simulink model "IK_Six_DOF_assembly2"  (R2022b)
settings: Solver=VariableStepAuto  StartTime=0.0  StopTime=500  RelTol=1e-3
model workspace: external: MATLAB File S:\project works\FYP\matlab\test2\6_DOF_assembly2\Assembly11_DataFile.m (data not in the file)
undefined symbols (not defined in the file or in its folder): sigbuilder_block, smiData, X, Y, Z
libraries: sm_lib x411, nesl_utility x45, slpidlib x14, robotcorelib x5, robotmaniplib x2
(part 2 of 9)

== system IK_Six_DOF_assembly2/Robot ==
  motion : Inport
  Calf Support Subsystem : Subsystem
  Initializer : Subsystem
  Subsystem : Subsystem
  Thigh/Slider Subsystem1 : Subsystem
  Thigh/Slider Subsystem2 : Subsystem
  qm : Outport
  wires:
  motion/1 -> Subsystem/1(motion)
  Subsystem/1(Position) -> qm/1  "qm"
  connections:
  Thigh/Slider Subsystem1/RConn1 -- Initializer/RConn1
  Calf Support Subsystem/LConn2 -- Thigh/Slider Subsystem2/LConn1
  Calf Support Subsystem/LConn1 -- Thigh/Slider Subsystem1/LConn1
  Subsystem/LConn1 -- Calf Support Subsystem/RConn1
  Subsystem/LConn2 -- Calf Support Subsystem/RConn2

== system IK_Six_DOF_assembly2/Robot1 ==
  torque : Inport
  Calf Support Subsystem : Subsystem
  Initializer : Subsystem
  Subsystem : Subsystem
  Thigh/Slider Subsystem1 : Subsystem
  Thigh/Slider Subsystem2 : Subsystem
  qm : Outport
  wires:
  Subsystem/1(Position) -> qm/1  "qm"
  torque/1 -> Subsystem/1(torque)
  connections:
  Subsystem/LConn2 -- Calf Support Subsystem/RConn2
  Subsystem/LConn1 -- Calf Support Subsystem/RConn1
  Calf Support Subsystem/LConn1 -- Thigh/Slider Subsystem1/LConn1
  Calf Support Subsystem/LConn2 -- Thigh/Slider Subsystem2/LConn1
  Thigh/Slider Subsystem1/RConn1 -- Initializer/RConn1

== system IK_Six_DOF_assembly2/Robot2 ==
  torque : Inport
  Calf Support Subsystem : Subsystem
  Initializer : Subsystem
  Subsystem : Subsystem
  Thigh/Slider Subsystem1 : Subsystem
  Thigh/Slider Subsystem2 : Subsystem
  qm : Outport
  wires:
  torque/1 -> Subsystem/1(torque)
  Subsystem/1(Position) -> qm/1  "qm"
  connections:
  Thigh/Slider Subsystem1/RConn1 -- Initializer/RConn1
  Calf Support Subsystem/LConn2 -- Thigh/Slider Subsystem2/LConn1
  Calf Support Subsystem/LConn1 -- Thigh/Slider Subsystem1/LConn1
  Subsystem/LConn1 -- Calf Support Subsystem/RConn1
  Subsystem/LConn2 -- Calf Support Subsystem/RConn2

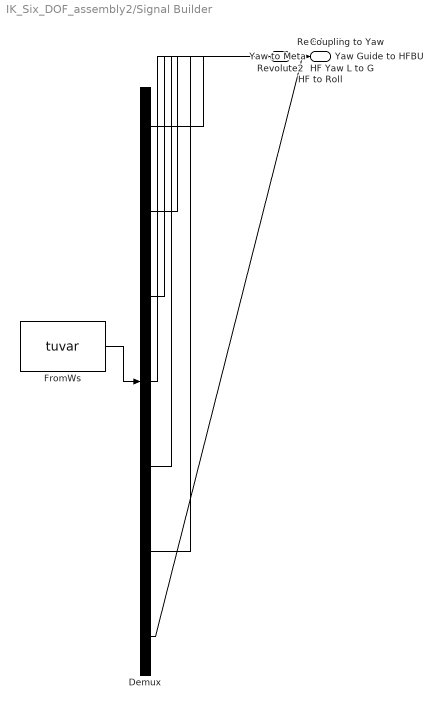
== system IK_Six_DOF_assembly2/Signal Builder ==
  Demux : Demux  Tag=STV Demux  Outputs=7
      settings: DisplayOption=none
  FromWs : FromWorkspace  Tag=STV FromWs  VariableName=tuvar
      SigBuilderData=|
      | common.afterFinalStr = 'Extrapolate'
      | common.sampleTime = 0
      | dataSet.timeRange = [0 10]
      | dataSet.name = 'Group 1'
      | sbobj.Groups.Name = 'Group 1'
      | sbobj.Groups.Signals(1).Name = 'Revolute2'
      | sbobj.Groups.Signals(1).XData = [0 3.5 3.5 6.52 6.52 10]
      | sbobj.Groups.Signals(1).YData = [0 0 0.4 0.4 0 0]
      | sbobj.Groups.Signals(2).Name = 'Revolute1'
      | sbobj.Groups.Signals(2).XData = [0 2.98 2.98 6.98 6.98 10]
      | sbobj.Groups.Signals(2).YData = [0 0 0.45 0.45 0 0]
      | sbobj.Groups.Signals(3).Name = 'HF Yaw L to G'
      | sbobj.Groups.Signals(3).XData = [0 2.5 2.5 7.62 7.62 10]
      | sbobj.Groups.Signals(3).YData = [0 0 0.3 0.3 0 0]
      | sbobj.Groups.Signals(4).Name = 'Yaw Guide to HFBU'
      | sbobj.Groups.Signals(4).XData = [0 2 2 8 8 10]
      | sbobj.Groups.Signals(4).YData = [0 0 0.4 0.4 0 0]
      | sbobj.Groups.Signals(5).Name = 'HF to Roll'
      | sbobj.Groups.Signals(5).XData = [0 1.46 1.46 8.6 8.6 10]
      | sbobj.Groups.Signals(5).YData = [0 0 0.35 0.35 0 0]
      | sbobj.Groups.Signals(6).Name = 'Yaw to Meta'
      | sbobj.Groups.Signals(6).XData = [0 1.02 1.02 9.04 9.04 10]
      | sbobj.Groups.Signals(6).YData = [0 0 0.2 0.2 0 0]
      | sbobj.Groups.Signals(7).Name = 'Coupling to Yaw'
      | sbobj.Groups.Signals(7).XData = [0 0.58 0.58 9.5 9.5 10]
      | sbobj.Groups.Signals(7).YData = [0 0 0.5 0.5 0 0]
  Revolute2 : Outport  Tag=STV Outport
  Revolute1 : Outport  Tag=STV Outport  Port=2
  HF Yaw L to G : Outport  Tag=STV Outport  Port=3
  Yaw Guide to HFBU : Outport  Tag=STV Outport  Port=4
  HF to Roll : Outport  Tag=STV Outport  Port=5
  Yaw to Meta : Outport  Tag=STV Outport  Port=6
  Coupling to Yaw : Outport  Tag=STV Outport  Port=7
  wires:
  FromWs/1 -> Demux/1
  Demux/1 -> Revolute2/1
  Demux/2 -> Revolute1/1
  Demux/3 -> HF Yaw L to G/1
  Demux/4 -> Yaw Guide to HFBU/1
  Demux/5 -> HF to Roll/1
  Demux/6 -> Yaw to Meta/1
  Demux/7 -> Coupling to Yaw/1

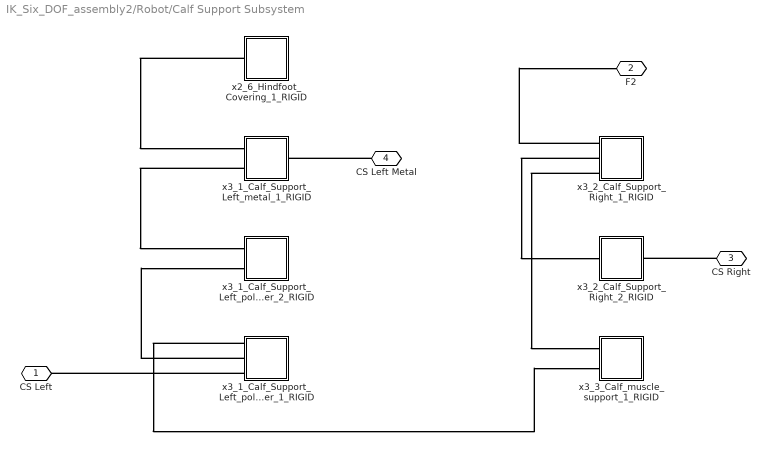
== system IK_Six_DOF_assembly2/Robot/Calf Support Subsystem ==
  x2_6_Hindfoot_Covering_1_RIGID : Subsystem
  x3_1_Calf_Support_Left_metal_1_RIGID : Subsystem
  x3_1_Calf_Support_Left_poly_upper_1_RIGID : Subsystem
  x3_1_Calf_Support_Left_poly_upper_2_RIGID : Subsystem
  x3_2_Calf_Support_Right_1_RIGID : Subsystem
  x3_2_Calf_Support_Right_2_RIGID : Subsystem
  x3_3_Calf_muscle_support_1_RIGID : Subsystem
  "CS Left " : PMIOPort  Side=Left
  F2 : PMIOPort  Port=2  Side=Left
  CS Right : PMIOPort  Port=3  Side=Right
  CS Left Metal : PMIOPort  Port=4  Side=Right
  connections:
  x2_6_Hindfoot_Covering_1_RIGID/LConn1 -- x3_1_Calf_Support_Left_metal_1_RIGID/LConn1
  x3_2_Calf_Support_Right_1_RIGID/LConn1 -- F2/RConn1
  x3_1_Calf_Support_Left_poly_upper_1_RIGID/LConn1 -- x3_3_Calf_muscle_support_1_RIGID/LConn2
  x3_2_Calf_Support_Right_1_RIGID/LConn2 -- x3_2_Calf_Support_Right_2_RIGID/LConn1
  CS Left Metal/RConn1 -- x3_1_Calf_Support_Left_metal_1_RIGID/RConn1
  x3_1_Calf_Support_Left_metal_1_RIGID/LConn2 -- x3_1_Calf_Support_Left_poly_upper_2_RIGID/LConn1
  x3_2_Calf_Support_Right_1_RIGID/LConn3 -- x3_3_Calf_muscle_support_1_RIGID/LConn1
  x3_1_Calf_Support_Left_poly_upper_1_RIGID/LConn2 -- x3_1_Calf_Support_Left_poly_upper_2_RIGID/LConn2
  CS Right/RConn1 -- x3_2_Calf_Support_Right_2_RIGID/RConn1
  x3_1_Calf_Support_Left_poly_upper_1_RIGID/LConn3 -- "CS Left "/RConn1

== system IK_Six_DOF_assembly2/Robot/Initializer ==
  MechanismConfiguration : sm_lib/Utilities/Mechanism Configuration  UniformGravity=Constant  GravityVector=[0 0 -9.80665]  GravityUnits=m/s^2  LinearizationDelta=0.001  JointModeTransitionNonlinearIterations=2
  Solver Configuration : nesl_utility/Solver Configuration  PhysicalDomain=network_engine_domain  SubClassName=solver  LeftPortType=input  RightPortType=generic  Tones=[]  Harmonics=[]  SimulateNoise=off  Profile=off  UseLocalSampling=off  EnableSwitchedLinearOptims=on  FrequencyDomain=off  UseCCode=off  RelTol=0.001  AbsTol=1e-06  MinStep=1e-09  ToWorkspace=off  RevertToSquareIcSolve=off  NumHomotopyIterations=100  PhasorMode=off  PhasorModeNumHarmonics=1  ConsistencySolver=NEWTON_FTOL  IndexReductionMethod=DerivativeReplacement  DoDC=off  ResidualTolerance=1e-09  ConsistencyTolSource=GLOBAL  ConsistencyAbsTol=0.001  ConsistencyRelTol=0.001  ConsistencyTolFactor=0.001  UseLocalSolver=off  LocalSolverChoice=NE_BACKWARD_EULER_ADVANCER  ResolveIndetEquations=on  FunctionEvalNumThread=1  LocalSolverSampleTime=0.001  DoFixedCost=off  MaxNonlinIter=3  MaxModeIter=2  ComputeImpulses=off  ImpulseIterations=2  LinearAlgebra=auto  LinearAlgebraNumThread=0  EquationFormulation=NE_TIME_EF  DelaysMemoryBudget=1024  AutomaticFiltering=on  FilteringTimeConstant=0.001  PartitionStorageMethod=AS_NEEDED  PartitionMemoryBudget=1024  PartitionMethod=ROBUST
  Transform : sm_lib/Frames and Transforms/Rigid Transform  TranslationMethod=Cartesian  TranslationStandardOffset=0  TranslationLengthUnit=in  TranslationStandardAxis=+Z  TranslationCartesianOffset=smiData.RigidTransform(63).translation  TranslationROffset=0  TranslationROffsetUnits=m  TranslationZOffset=0  TranslationZOffsetUnits=m  TranslationThetaOffset=0  TranslationThetaOffsetUnits=deg  RotationMethod=ArbitraryAxis  RotationAngleUnits=rad  RotationStandardAxis=+Z  RotationAngle=smiData.RigidTransform(63).angle  RotationArbitraryAxis=smiData.RigidTransform(63).axis  FollAlignAxisA=+X  BaseAlignAxisA=+Y  FollAlignAxisB=+Y  BaseAlignAxisB=+Z  RotationSequenceAxes=FollowerAxes  RotationSequence=XYX  RotationSequenceAngles=[0 0 0]  RotationSequenceAnglesUnits=deg  RotationMatrix=[1 0 0; 0 1 0; 0 0 1]  Quaternion=[1 0 0 0]
  World : sm_lib/Frames and Transforms/World Frame
  F2 : PMIOPort  Side=Right
  connections:
  Transform/LConn1 -- Solver Configuration/RConn1 -- MechanismConfiguration/RConn1 -- World/RConn1
  Transform/RConn1 -- F2/RConn1

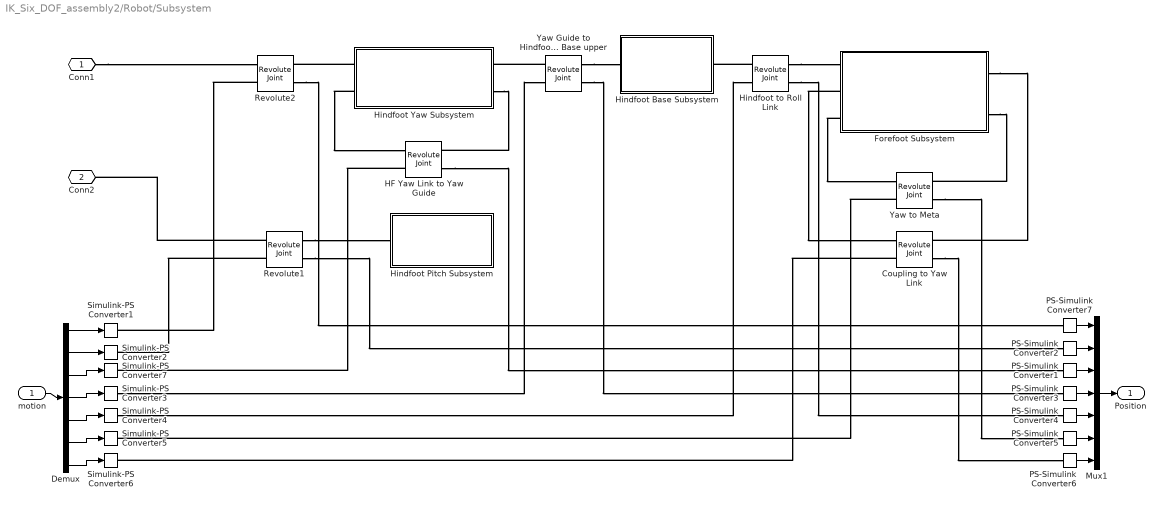
== system IK_Six_DOF_assembly2/Robot/Subsystem ==
  motion : Inport
  Coupling to Yaw Link : sm_lib/Joints/Revolute Joint  JointMode=Normal  SenseConstraintForce=off  SenseConstraintForceX=off  SenseConstraintForceY=off  SenseConstraintForceZ=off  SenseConstraintTorque=off  SenseConstraintTorqueX=off  SenseConstraintTorqueY=off  SenseConstraintTorqueZ=off  SenseTotalForce=off  SenseTotalForceX=off  SenseTotalForceY=off  SenseTotalForceZ=off  SenseTotalTorque=off  SenseTotalTorqueX=off  SenseTotalTorqueY=off  SenseTotalTorqueZ=off  CompositeWrenchDir=FollowerOnBase  CompositeWrenchFrame=BaseFrame  EquilibriumPosition=0  EquilibriumPositionUnits=deg  SpringStiffness=0  SpringStiffnessUnits=N*m/deg  DampingCoefficient=0  DampingCoefficientUnits=N*m/(deg/s)  TorqueActuationMode=ComputedTorque  MotionActuationMode=InputMotion  SensePosition=on  SenseVelocity=off  SenseAcceleration=off  SenseTorqueForce=off  SenseLowerLimitTorqueForce=off  SenseUpperLimitTorqueForce=off  LowerLimitSpecify=off  LowerLimitBound=-90  LowerLimitBoundUnits=deg  LowerLimitStiffness=1e4  LowerLimitStiffnessUnits=N*m/deg  LowerLimitDamping=10  LowerLimitDampingUnits=N*m/(deg/s)  LowerLimitTransitionRegionWidth=0.1  LowerLimitTransitionRegionWidthUnits=deg  UpperLimitSpecify=off  UpperLimitBound=90  UpperLimitBoundUnits=deg  UpperLimitStiffness=1e4  UpperLimitStiffnessUnits=N*m/deg  UpperLimitDamping=10  UpperLimitDampingUnits=N*m/(deg/s)  UpperLimitTransitionRegionWidth=0.1  UpperLimitTransitionRegionWidthUnits=deg  PositionTargetSpecify=on  PositionTargetPriority=Low  PositionTargetValue=smiData.RevoluteJoint(7).Rz.Pos  PositionTargetValueUnits=deg  VelocityTargetSpecify=off  VelocityTargetPriority=High  VelocityTargetValue=0  VelocityTargetValueUnits=deg/s
  Demux : Demux  Outputs=7
  Forefoot Subsystem : Subsystem
  HF Yaw Link to Yaw Guide : sm_lib/Joints/Revolute Joint  JointMode=Normal  SenseConstraintForce=off  SenseConstraintForceX=off  SenseConstraintForceY=off  SenseConstraintForceZ=off  SenseConstraintTorque=off  SenseConstraintTorqueX=off  SenseConstraintTorqueY=off  SenseConstraintTorqueZ=off  SenseTotalForce=off  SenseTotalForceX=off  SenseTotalForceY=off  SenseTotalForceZ=off  SenseTotalTorque=off  SenseTotalTorqueX=off  SenseTotalTorqueY=off  SenseTotalTorqueZ=off  CompositeWrenchDir=FollowerOnBase  CompositeWrenchFrame=BaseFrame  EquilibriumPosition=0  EquilibriumPositionUnits=deg  SpringStiffness=0  SpringStiffnessUnits=N*m/deg  DampingCoefficient=0  DampingCoefficientUnits=N*m/(deg/s)  TorqueActuationMode=ComputedTorque  MotionActuationMode=InputMotion  SensePosition=on  SenseVelocity=off  SenseAcceleration=off  SenseTorqueForce=off  SenseLowerLimitTorqueForce=off  SenseUpperLimitTorqueForce=off  LowerLimitSpecify=off  LowerLimitBound=-30  LowerLimitBoundUnits=deg  LowerLimitStiffness=1e4  LowerLimitStiffnessUnits=N*m/deg  LowerLimitDamping=10  LowerLimitDampingUnits=N*m/(deg/s)  LowerLimitTransitionRegionWidth=0.1  LowerLimitTransitionRegionWidthUnits=deg  UpperLimitSpecify=off  UpperLimitBound=30  UpperLimitBoundUnits=deg  UpperLimitStiffness=1e4  UpperLimitStiffnessUnits=N*m/deg  UpperLimitDamping=10  UpperLimitDampingUnits=N*m/(deg/s)  UpperLimitTransitionRegionWidth=0.1  UpperLimitTransitionRegionWidthUnits=deg  PositionTargetSpecify=on  PositionTargetPriority=Low  PositionTargetValue=smiData.RevoluteJoint(2).Rz.Pos  PositionTargetValueUnits=deg  VelocityTargetSpecify=off  VelocityTargetPriority=High  VelocityTargetValue=0  VelocityTargetValueUnits=deg/s
  Hindfoot Base Subsystem : Subsystem
  Hindfoot Pitch Subsystem : Subsystem
  Hindfoot Yaw Subsystem : Subsystem
  Hindfoot to Roll Link : sm_lib/Joints/Revolute Joint  JointMode=Normal  SenseConstraintForce=off  SenseConstraintForceX=off  SenseConstraintForceY=off  SenseConstraintForceZ=off  SenseConstraintTorque=off  SenseConstraintTorqueX=off  SenseConstraintTorqueY=off  SenseConstraintTorqueZ=off  SenseTotalForce=off  SenseTotalForceX=off  SenseTotalForceY=off  SenseTotalForceZ=off  SenseTotalTorque=off  SenseTotalTorqueX=off  SenseTotalTorqueY=off  SenseTotalTorqueZ=off  CompositeWrenchDir=FollowerOnBase  CompositeWrenchFrame=BaseFrame  EquilibriumPosition=0  EquilibriumPositionUnits=deg  SpringStiffness=0  SpringStiffnessUnits=N*m/deg  DampingCoefficient=0  DampingCoefficientUnits=N*m/(deg/s)  TorqueActuationMode=ComputedTorque  MotionActuationMode=InputMotion  SensePosition=on  SenseVelocity=off  SenseAcceleration=off  SenseTorqueForce=off  SenseLowerLimitTorqueForce=off  SenseUpperLimitTorqueForce=off  LowerLimitSpecify=off  LowerLimitBound=-90  LowerLimitBoundUnits=deg  LowerLimitStiffness=1e4  LowerLimitStiffnessUnits=N*m/deg  LowerLimitDamping=10  LowerLimitDampingUnits=N*m/(deg/s)  LowerLimitTransitionRegionWidth=0.1  LowerLimitTransitionRegionWidthUnits=deg  UpperLimitSpecify=off  UpperLimitBound=90  UpperLimitBoundUnits=deg  UpperLimitStiffness=1e4  UpperLimitStiffnessUnits=N*m/deg  UpperLimitDamping=10  UpperLimitDampingUnits=N*m/(deg/s)  UpperLimitTransitionRegionWidth=0.1  UpperLimitTransitionRegionWidthUnits=deg  PositionTargetSpecify=on  PositionTargetPriority=Low  PositionTargetValue=smiData.RevoluteJoint(6).Rz.Pos  PositionTargetValueUnits=deg  VelocityTargetSpecify=off  VelocityTargetPriority=High  VelocityTargetValue=0  VelocityTargetValueUnits=deg/s
  Mux1 : Mux  Inputs=7
  PS-Simulink Converter{1..7} (7 alike) : nesl_utility/PS-Simulink Converter  PhysicalDomain=network_engine_domain  SubClassName=ps_output  LeftPortType=input  RightPortType=output  PseudoPeriodic=off  Frequencies=[]  VectorFormat=1-D array  Unit=inherit  AffineConversion=off
  Revolute1 : sm_lib/Joints/Revolute Joint  JointMode=Normal  SenseConstraintForce=off  SenseConstraintForceX=off  SenseConstraintForceY=off  SenseConstraintForceZ=off  SenseConstraintTorque=off  SenseConstraintTorqueX=off  SenseConstraintTorqueY=off  SenseConstraintTorqueZ=off  SenseTotalForce=off  SenseTotalForceX=off  SenseTotalForceY=off  SenseTotalForceZ=off  SenseTotalTorque=off  SenseTotalTorqueX=off  SenseTotalTorqueY=off  SenseTotalTorqueZ=off  CompositeWrenchDir=FollowerOnBase  CompositeWrenchFrame=BaseFrame  EquilibriumPosition=0  EquilibriumPositionUnits=deg  SpringStiffness=0  SpringStiffnessUnits=N*m/deg  DampingCoefficient=0  DampingCoefficientUnits=N*m/(deg/s)  TorqueActuationMode=ComputedTorque  MotionActuationMode=InputMotion  SensePosition=on  SenseVelocity=off  SenseAcceleration=off  SenseTorqueForce=off  SenseLowerLimitTorqueForce=off  SenseUpperLimitTorqueForce=off  LowerLimitSpecify=off  LowerLimitBound=-25  LowerLimitBoundUnits=deg  LowerLimitStiffness=1e4  LowerLimitStiffnessUnits=N*m/deg  LowerLimitDamping=10  LowerLimitDampingUnits=N*m/(deg/s)  LowerLimitTransitionRegionWidth=0.1  LowerLimitTransitionRegionWidthUnits=deg  UpperLimitSpecify=off  UpperLimitBound=25  UpperLimitBoundUnits=deg  UpperLimitStiffness=1e4  UpperLimitStiffnessUnits=N*m/deg  UpperLimitDamping=10  UpperLimitDampingUnits=N*m/(deg/s)  UpperLimitTransitionRegionWidth=0.1  UpperLimitTransitionRegionWidthUnits=deg  PositionTargetSpecify=on  PositionTargetPriority=Low  PositionTargetValue=smiData.RevoluteJoint(4).Rz.Pos  PositionTargetValueUnits=deg  VelocityTargetSpecify=off  VelocityTargetPriority=High  VelocityTargetValue=0  VelocityTargetValueUnits=deg/s
  Revolute2 : sm_lib/Joints/Revolute Joint  JointMode=Normal  SenseConstraintForce=off  SenseConstraintForceX=off  SenseConstraintForceY=off  SenseConstraintForceZ=off  SenseConstraintTorque=off  SenseConstraintTorqueX=off  SenseConstraintTorqueY=off  SenseConstraintTorqueZ=off  SenseTotalForce=off  SenseTotalForceX=off  SenseTotalForceY=off  SenseTotalForceZ=off  SenseTotalTorque=off  SenseTotalTorqueX=off  SenseTotalTorqueY=off  SenseTotalTorqueZ=off  CompositeWrenchDir=FollowerOnBase  CompositeWrenchFrame=BaseFrame  EquilibriumPosition=0  EquilibriumPositionUnits=deg  SpringStiffness=0  SpringStiffnessUnits=N*m/deg  DampingCoefficient=0  DampingCoefficientUnits=N*m/(deg/s)  TorqueActuationMode=ComputedTorque  MotionActuationMode=InputMotion  SensePosition=on  SenseVelocity=off  SenseAcceleration=off  SenseTorqueForce=off  SenseLowerLimitTorqueForce=off  SenseUpperLimitTorqueForce=off  LowerLimitSpecify=off  LowerLimitBound=-25  LowerLimitBoundUnits=deg  LowerLimitStiffness=1e4  LowerLimitStiffnessUnits=N*m/deg  LowerLimitDamping=10  LowerLimitDampingUnits=N*m/(deg/s)  LowerLimitTransitionRegionWidth=0.1  LowerLimitTransitionRegionWidthUnits=deg  UpperLimitSpecify=off  UpperLimitBound=25  UpperLimitBoundUnits=deg  UpperLimitStiffness=1e4  UpperLimitStiffnessUnits=N*m/deg  UpperLimitDamping=10  UpperLimitDampingUnits=N*m/(deg/s)  UpperLimitTransitionRegionWidth=0.1  UpperLimitTransitionRegionWidthUnits=deg  PositionTargetSpecify=on  PositionTargetPriority=Low  PositionTargetValue=smiData.RevoluteJoint(4).Rz.Pos  PositionTargetValueUnits=deg  VelocityTargetSpecify=off  VelocityTargetPriority=High  VelocityTargetValue=0  VelocityTargetValueUnits=deg/s
  Simulink-PS Converter{1..7} (7 alike) : nesl_utility/Simulink-PS Converter  PhysicalDomain=network_engine_domain  SubClassName=ps_input  LeftPortType=input  RightPortType=output  PseudoPeriodic=off  Frequencies=[]  NoiseDistribution=none  NoiseParameters=[]  Unit=rad  AffineConversion=off  FilteringAndDerivatives=filter  SimscapeFilterOrder=2  InputFilterTimeConstant=0.001  UdotUserProvided=0
  Yaw Guide to Hindfoot Base upper : sm_lib/Joints/Revolute Joint  JointMode=Normal  SenseConstraintForce=off  SenseConstraintForceX=off  SenseConstraintForceY=off  SenseConstraintForceZ=off  SenseConstraintTorque=off  SenseConstraintTorqueX=off  SenseConstraintTorqueY=off  SenseConstraintTorqueZ=off  SenseTotalForce=off  SenseTotalForceX=off  SenseTotalForceY=off  SenseTotalForceZ=off  SenseTotalTorque=off  SenseTotalTorqueX=off  SenseTotalTorqueY=off  SenseTotalTorqueZ=off  CompositeWrenchDir=FollowerOnBase  CompositeWrenchFrame=BaseFrame  EquilibriumPosition=0  EquilibriumPositionUnits=deg  SpringStiffness=0  SpringStiffnessUnits=N*m/deg  DampingCoefficient=0  DampingCoefficientUnits=N*m/(deg/s)  TorqueActuationMode=ComputedTorque  MotionActuationMode=InputMotion  SensePosition=on  SenseVelocity=off  SenseAcceleration=off  SenseTorqueForce=off  SenseLowerLimitTorqueForce=off  SenseUpperLimitTorqueForce=off  LowerLimitSpecify=off  LowerLimitBound=-90  LowerLimitBoundUnits=deg  LowerLimitStiffness=1e4  LowerLimitStiffnessUnits=N*m/deg  LowerLimitDamping=10  LowerLimitDampingUnits=N*m/(deg/s)  LowerLimitTransitionRegionWidth=0.1  LowerLimitTransitionRegionWidthUnits=deg  UpperLimitSpecify=off  UpperLimitBound=90  UpperLimitBoundUnits=deg  UpperLimitStiffness=1e4  UpperLimitStiffnessUnits=N*m/deg  UpperLimitDamping=10  UpperLimitDampingUnits=N*m/(deg/s)  UpperLimitTransitionRegionWidth=0.1  UpperLimitTransitionRegionWidthUnits=deg  PositionTargetSpecify=on  PositionTargetPriority=Low  PositionTargetValue=smiData.RevoluteJoint(3).Rz.Pos  PositionTargetValueUnits=deg  VelocityTargetSpecify=off  VelocityTargetPriority=High  VelocityTargetValue=0  VelocityTargetValueUnits=deg/s
  Yaw to Meta : sm_lib/Joints/Revolute Joint  JointMode=Normal  SenseConstraintForce=off  SenseConstraintForceX=off  SenseConstraintForceY=off  SenseConstraintForceZ=off  SenseConstraintTorque=off  SenseConstraintTorqueX=off  SenseConstraintTorqueY=off  SenseConstraintTorqueZ=off  SenseTotalForce=off  SenseTotalForceX=off  SenseTotalForceY=off  SenseTotalForceZ=off  SenseTotalTorque=off  SenseTotalTorqueX=off  SenseTotalTorqueY=off  SenseTotalTorqueZ=off  CompositeWrenchDir=FollowerOnBase  CompositeWrenchFrame=BaseFrame  EquilibriumPosition=0  EquilibriumPositionUnits=deg  SpringStiffness=0  SpringStiffnessUnits=N*m/deg  DampingCoefficient=0  DampingCoefficientUnits=N*m/(deg/s)  TorqueActuationMode=ComputedTorque  MotionActuationMode=InputMotion  SensePosition=on  SenseVelocity=off  SenseAcceleration=off  SenseTorqueForce=off  SenseLowerLimitTorqueForce=off  SenseUpperLimitTorqueForce=off  LowerLimitSpecify=off  LowerLimitBound=-90  LowerLimitBoundUnits=deg  LowerLimitStiffness=1e4  LowerLimitStiffnessUnits=N*m/deg  LowerLimitDamping=10  LowerLimitDampingUnits=N*m/(deg/s)  LowerLimitTransitionRegionWidth=0.1  LowerLimitTransitionRegionWidthUnits=deg  UpperLimitSpecify=off  UpperLimitBound=90  UpperLimitBoundUnits=deg  UpperLimitStiffness=1e4  UpperLimitStiffnessUnits=N*m/deg  UpperLimitDamping=10  UpperLimitDampingUnits=N*m/(deg/s)  UpperLimitTransitionRegionWidth=0.1  UpperLimitTransitionRegionWidthUnits=deg  PositionTargetSpecify=on  PositionTargetPriority=Low  PositionTargetValue=smiData.RevoluteJoint(5).Rz.Pos  PositionTargetValueUnits=deg  VelocityTargetSpecify=off  VelocityTargetPriority=High  VelocityTargetValue=0  VelocityTargetValueUnits=deg/s
  Conn1 : PMIOPort  Side=Left
  Conn2 : PMIOPort  Port=2  Side=Left
  Position : Outport
  wires:
  motion/1 -> Demux/1
  Demux/6 -> Simulink-PS Converter5/1
  Mux1/1 -> Position/1
  Demux/5 -> Simulink-PS Converter4/1
  Demux/7 -> Simulink-PS Converter6/1
  Demux/4 -> Simulink-PS Converter3/1
  PS-Simulink Converter3/1 -> Mux1/4
  PS-Simulink Converter4/1 -> Mux1/5
  PS-Simulink Converter5/1 -> Mux1/6
  PS-Simulink Converter6/1 -> Mux1/7
  Demux/1 -> Simulink-PS Converter1/1
  Demux/2 -> Simulink-PS Converter2/1
  Demux/3 -> Simulink-PS Converter7/1
  PS-Simulink Converter7/1 -> Mux1/1
  PS-Simulink Converter2/1 -> Mux1/2
  PS-Simulink Converter1/1 -> Mux1/3
  connections:
  Yaw Guide to Hindfoot Base upper/LConn1 -- Hindfoot Yaw Subsystem/RConn1
  Yaw Guide to Hindfoot Base upper/RConn1 -- Hindfoot Base Subsystem/LConn1
  Hindfoot to Roll Link/RConn2 -- PS-Simulink Converter4/LConn1
  Hindfoot to Roll Link/LConn1 -- Hindfoot Base Subsystem/RConn1
  Hindfoot to Roll Link/RConn1 -- Forefoot Subsystem/LConn1
  Revolute1/RConn1 -- Hindfoot Pitch Subsystem/LConn1
  Conn1/RConn1 -- Revolute2/LConn1
  Hindfoot Yaw Subsystem/RConn2 -- HF Yaw Link to Yaw Guide/RConn1
  Hindfoot Yaw Subsystem/LConn2 -- HF Yaw Link to Yaw Guide/LConn1
  Forefoot Subsystem/RConn2 -- Yaw to Meta/RConn1
  Yaw to Meta/LConn2 -- Simulink-PS Converter5/RConn1
  Forefoot Subsystem/LConn2 -- Coupling to Yaw Link/LConn1
  Revolute1/LConn1 -- Conn2/RConn1
  Coupling to Yaw Link/LConn2 -- Simulink-PS Converter6/RConn1
  Coupling to Yaw Link/RConn2 -- PS-Simulink Converter6/LConn1
  Yaw to Meta/RConn2 -- PS-Simulink Converter5/LConn1
  Simulink-PS Converter4/RConn1 -- Hindfoot to Roll Link/LConn2
  Forefoot Subsystem/RConn1 -- Coupling to Yaw Link/RConn1
  Forefoot Subsystem/LConn3 -- Yaw to Meta/LConn1
  Yaw Guide to Hindfoot Base upper/RConn2 -- PS-Simulink Converter3/LConn1
  Simulink-PS Converter3/RConn1 -- Yaw Guide to Hindfoot Base upper/LConn2
  Hindfoot Yaw Subsystem/LConn1 -- Revolute2/RConn1
  Revolute2/LConn2 -- Simulink-PS Converter1/RConn1
  Revolute1/LConn2 -- Simulink-PS Converter2/RConn1
  HF Yaw Link to Yaw Guide/LConn2 -- Simulink-PS Converter7/RConn1
  Revolute2/RConn2 -- PS-Simulink Converter7/LConn1
  Revolute1/RConn2 -- PS-Simulink Converter2/LConn1
  HF Yaw Link to Yaw Guide/RConn2 -- PS-Simulink Converter1/LConn1

== system IK_Six_DOF_assembly2/Robot/Thigh//Slider Subsystem1 ==
  x4_1_Slider_Link_1_RIGID : Subsystem
  x4_3_Thigh_Link_1_RIGID : Subsystem
  F1 : PMIOPort  Side=Left
  F2 : PMIOPort  Port=2  Side=Right
  connections:
  x4_1_Slider_Link_1_RIGID/LConn3 -- x4_3_Thigh_Link_1_RIGID/LConn1
  F1/RConn1 -- x4_1_Slider_Link_1_RIGID/LConn1
  F2/RConn1 -- x4_1_Slider_Link_1_RIGID/LConn2

== system IK_Six_DOF_assembly2/Robot/Thigh//Slider Subsystem2 ==
  x4_1_Slider_Link_2_RIGID : Subsystem
  x4_3_Thigh_Link_2_RIGID : Subsystem
  F : PMIOPort  Side=Left
  connections:
  x4_1_Slider_Link_2_RIGID/LConn1 -- x4_3_Thigh_Link_2_RIGID/LConn1
  F/RConn1 -- x4_1_Slider_Link_2_RIGID/LConn2

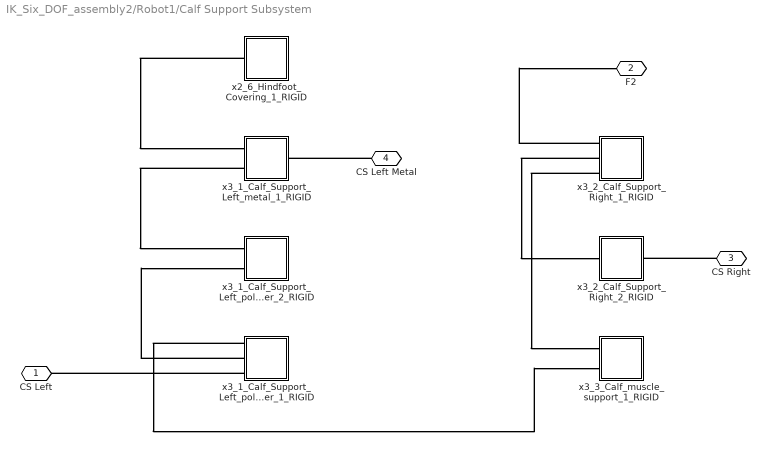
== system IK_Six_DOF_assembly2/Robot1/Calf Support Subsystem ==
  x2_6_Hindfoot_Covering_1_RIGID : Subsystem
  x3_1_Calf_Support_Left_metal_1_RIGID : Subsystem
  x3_1_Calf_Support_Left_poly_upper_1_RIGID : Subsystem
  x3_1_Calf_Support_Left_poly_upper_2_RIGID : Subsystem
  x3_2_Calf_Support_Right_1_RIGID : Subsystem
  x3_2_Calf_Support_Right_2_RIGID : Subsystem
  x3_3_Calf_muscle_support_1_RIGID : Subsystem
  "CS Left " : PMIOPort  Side=Left
  F2 : PMIOPort  Port=2  Side=Left
  CS Right : PMIOPort  Port=3  Side=Right
  CS Left Metal : PMIOPort  Port=4  Side=Right
  connections:
  x3_1_Calf_Support_Left_poly_upper_1_RIGID/LConn3 -- "CS Left "/RConn1
  CS Right/RConn1 -- x3_2_Calf_Support_Right_2_RIGID/RConn1
  x3_1_Calf_Support_Left_poly_upper_1_RIGID/LConn2 -- x3_1_Calf_Support_Left_poly_upper_2_RIGID/LConn2
  x3_2_Calf_Support_Right_1_RIGID/LConn3 -- x3_3_Calf_muscle_support_1_RIGID/LConn1
  x3_1_Calf_Support_Left_metal_1_RIGID/LConn2 -- x3_1_Calf_Support_Left_poly_upper_2_RIGID/LConn1
  CS Left Metal/RConn1 -- x3_1_Calf_Support_Left_metal_1_RIGID/RConn1
  x3_2_Calf_Support_Right_1_RIGID/LConn2 -- x3_2_Calf_Support_Right_2_RIGID/LConn1
  x3_1_Calf_Support_Left_poly_upper_1_RIGID/LConn1 -- x3_3_Calf_muscle_support_1_RIGID/LConn2
  x3_2_Calf_Support_Right_1_RIGID/LConn1 -- F2/RConn1
  x2_6_Hindfoot_Covering_1_RIGID/LConn1 -- x3_1_Calf_Support_Left_metal_1_RIGID/LConn1

== system IK_Six_DOF_assembly2/Robot1/Initializer ==
  MechanismConfiguration : sm_lib/Utilities/Mechanism Configuration  UniformGravity=Constant  GravityVector=[0 0 -9.80665]  GravityUnits=m/s^2  LinearizationDelta=0.001  JointModeTransitionNonlinearIterations=2
  Solver Configuration : nesl_utility/Solver Configuration  PhysicalDomain=network_engine_domain  SubClassName=solver  LeftPortType=input  RightPortType=generic  Tones=[]  Harmonics=[]  SimulateNoise=off  Profile=off  UseLocalSampling=off  EnableSwitchedLinearOptims=on  FrequencyDomain=off  UseCCode=off  RelTol=0.001  AbsTol=1e-06  MinStep=1e-09  ToWorkspace=off  RevertToSquareIcSolve=off  NumHomotopyIterations=100  PhasorMode=off  PhasorModeNumHarmonics=1  ConsistencySolver=NEWTON_FTOL  IndexReductionMethod=DerivativeReplacement  DoDC=off  ResidualTolerance=1e-09  ConsistencyTolSource=GLOBAL  ConsistencyAbsTol=0.001  ConsistencyRelTol=0.001  ConsistencyTolFactor=0.001  UseLocalSolver=off  LocalSolverChoice=NE_BACKWARD_EULER_ADVANCER  ResolveIndetEquations=on  FunctionEvalNumThread=1  LocalSolverSampleTime=0.001  DoFixedCost=off  MaxNonlinIter=3  MaxModeIter=2  ComputeImpulses=off  ImpulseIterations=2  LinearAlgebra=auto  LinearAlgebraNumThread=0  EquationFormulation=NE_TIME_EF  DelaysMemoryBudget=1024  AutomaticFiltering=on  FilteringTimeConstant=0.001  PartitionStorageMethod=AS_NEEDED  PartitionMemoryBudget=1024  PartitionMethod=ROBUST
  Transform : sm_lib/Frames and Transforms/Rigid Transform  TranslationMethod=Cartesian  TranslationStandardOffset=0  TranslationLengthUnit=in  TranslationStandardAxis=+Z  TranslationCartesianOffset=smiData.RigidTransform(63).translation  TranslationROffset=0  TranslationROffsetUnits=m  TranslationZOffset=0  TranslationZOffsetUnits=m  TranslationThetaOffset=0  TranslationThetaOffsetUnits=deg  RotationMethod=ArbitraryAxis  RotationAngleUnits=rad  RotationStandardAxis=+Z  RotationAngle=smiData.RigidTransform(63).angle  RotationArbitraryAxis=smiData.RigidTransform(63).axis  FollAlignAxisA=+X  BaseAlignAxisA=+Y  FollAlignAxisB=+Y  BaseAlignAxisB=+Z  RotationSequenceAxes=FollowerAxes  RotationSequence=XYX  RotationSequenceAngles=[0 0 0]  RotationSequenceAnglesUnits=deg  RotationMatrix=[1 0 0; 0 1 0; 0 0 1]  Quaternion=[1 0 0 0]
  World : sm_lib/Frames and Transforms/World Frame
  F2 : PMIOPort  Side=Right
  connections:
  Transform/RConn1 -- F2/RConn1
  World/RConn1 -- MechanismConfiguration/RConn1 -- Solver Configuration/RConn1 -- Transform/LConn1

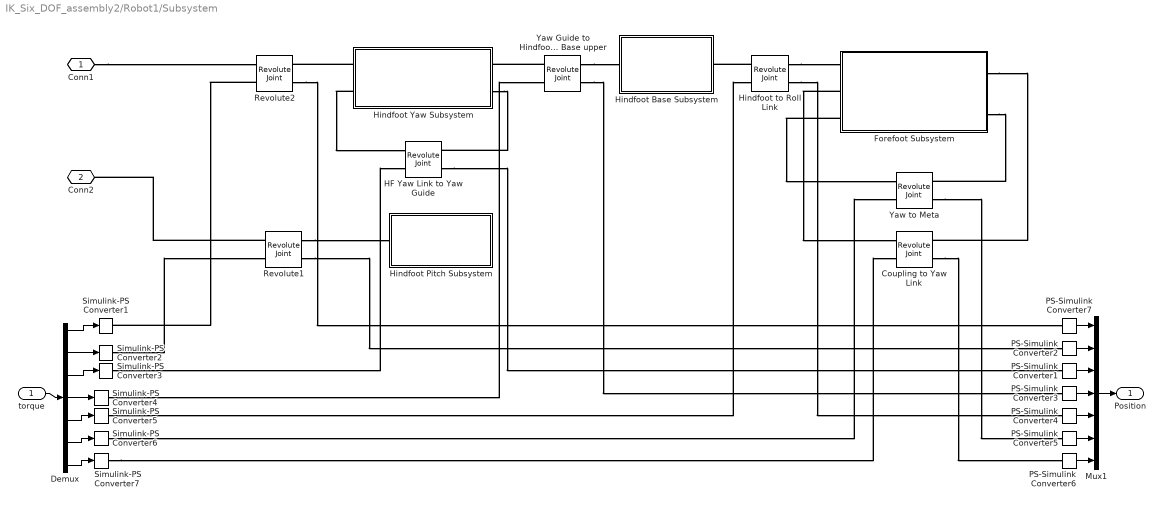
== system IK_Six_DOF_assembly2/Robot1/Subsystem ==
  torque : Inport
  Coupling to Yaw Link : sm_lib/Joints/Revolute Joint  JointMode=Normal  SenseConstraintForce=off  SenseConstraintForceX=off  SenseConstraintForceY=off  SenseConstraintForceZ=off  SenseConstraintTorque=off  SenseConstraintTorqueX=off  SenseConstraintTorqueY=off  SenseConstraintTorqueZ=off  SenseTotalForce=off  SenseTotalForceX=off  SenseTotalForceY=off  SenseTotalForceZ=off  SenseTotalTorque=off  SenseTotalTorqueX=off  SenseTotalTorqueY=off  SenseTotalTorqueZ=off  CompositeWrenchDir=FollowerOnBase  CompositeWrenchFrame=BaseFrame  EquilibriumPosition=0  EquilibriumPositionUnits=deg  SpringStiffness=0  SpringStiffnessUnits=N*m/deg  DampingCoefficient=0  DampingCoefficientUnits=N*m/(deg/s)  TorqueActuationMode=InputTorque  MotionActuationMode=ComputedMotion  SensePosition=on  SenseVelocity=off  SenseAcceleration=off  SenseTorqueForce=off  SenseLowerLimitTorqueForce=off  SenseUpperLimitTorqueForce=off  LowerLimitSpecify=on  LowerLimitBound=-25  LowerLimitBoundUnits=deg  LowerLimitStiffness=1e4  LowerLimitStiffnessUnits=N*m/deg  LowerLimitDamping=10  LowerLimitDampingUnits=N*m/(deg/s)  LowerLimitTransitionRegionWidth=0.1  LowerLimitTransitionRegionWidthUnits=deg  UpperLimitSpecify=on  UpperLimitBound=25  UpperLimitBoundUnits=deg  UpperLimitStiffness=1e4  UpperLimitStiffnessUnits=N*m/deg  UpperLimitDamping=10  UpperLimitDampingUnits=N*m/(deg/s)  UpperLimitTransitionRegionWidth=0.1  UpperLimitTransitionRegionWidthUnits=deg  PositionTargetSpecify=on  PositionTargetPriority=Low  PositionTargetValue=smiData.RevoluteJoint(7).Rz.Pos  PositionTargetValueUnits=deg  VelocityTargetSpecify=off  VelocityTargetPriority=High  VelocityTargetValue=0  VelocityTargetValueUnits=deg/s
  Demux : Demux  Outputs=7
  Forefoot Subsystem : Subsystem
  HF Yaw Link to Yaw Guide : sm_lib/Joints/Revolute Joint  JointMode=Normal  SenseConstraintForce=off  SenseConstraintForceX=off  SenseConstraintForceY=off  SenseConstraintForceZ=off  SenseConstraintTorque=off  SenseConstraintTorqueX=off  SenseConstraintTorqueY=off  SenseConstraintTorqueZ=off  SenseTotalForce=off  SenseTotalForceX=off  SenseTotalForceY=off  SenseTotalForceZ=off  SenseTotalTorque=off  SenseTotalTorqueX=off  SenseTotalTorqueY=off  SenseTotalTorqueZ=off  CompositeWrenchDir=FollowerOnBase  CompositeWrenchFrame=BaseFrame  EquilibriumPosition=0  EquilibriumPositionUnits=deg  SpringStiffness=0  SpringStiffnessUnits=N*m/deg  DampingCoefficient=0  DampingCoefficientUnits=N*m/(deg/s)  TorqueActuationMode=InputTorque  MotionActuationMode=ComputedMotion  SensePosition=on  SenseVelocity=off  SenseAcceleration=off  SenseTorqueForce=off  SenseLowerLimitTorqueForce=off  SenseUpperLimitTorqueForce=off  LowerLimitSpecify=on  LowerLimitBound=-30  LowerLimitBoundUnits=deg  LowerLimitStiffness=1e4  LowerLimitStiffnessUnits=N*m/deg  LowerLimitDamping=10  LowerLimitDampingUnits=N*m/(deg/s)  LowerLimitTransitionRegionWidth=0.1  LowerLimitTransitionRegionWidthUnits=deg  UpperLimitSpecify=on  UpperLimitBound=30  UpperLimitBoundUnits=deg  UpperLimitStiffness=1e4  UpperLimitStiffnessUnits=N*m/deg  UpperLimitDamping=10  UpperLimitDampingUnits=N*m/(deg/s)  UpperLimitTransitionRegionWidth=0.1  UpperLimitTransitionRegionWidthUnits=deg  PositionTargetSpecify=on  PositionTargetPriority=Low  PositionTargetValue=smiData.RevoluteJoint(2).Rz.Pos  PositionTargetValueUnits=deg  VelocityTargetSpecify=off  VelocityTargetPriority=High  VelocityTargetValue=0  VelocityTargetValueUnits=deg/s
  Hindfoot Base Subsystem : Subsystem
  Hindfoot Pitch Subsystem : Subsystem
  Hindfoot Yaw Subsystem : Subsystem
  Hindfoot to Roll Link : sm_lib/Joints/Revolute Joint  JointMode=Normal  SenseConstraintForce=off  SenseConstraintForceX=off  SenseConstraintForceY=off  SenseConstraintForceZ=off  SenseConstraintTorque=off  SenseConstraintTorqueX=off  SenseConstraintTorqueY=off  SenseConstraintTorqueZ=off  SenseTotalForce=off  SenseTotalForceX=off  SenseTotalForceY=off  SenseTotalForceZ=off  SenseTotalTorque=off  SenseTotalTorqueX=off  SenseTotalTorqueY=off  SenseTotalTorqueZ=off  CompositeWrenchDir=FollowerOnBase  CompositeWrenchFrame=BaseFrame  EquilibriumPosition=0  EquilibriumPositionUnits=deg  SpringStiffness=0  SpringStiffnessUnits=N*m/deg  DampingCoefficient=0  DampingCoefficientUnits=N*m/(deg/s)  TorqueActuationMode=InputTorque  MotionActuationMode=ComputedMotion  SensePosition=on  SenseVelocity=off  SenseAcceleration=off  SenseTorqueForce=off  SenseLowerLimitTorqueForce=off  SenseUpperLimitTorqueForce=off  LowerLimitSpecify=on  LowerLimitBound=-45  LowerLimitBoundUnits=deg  LowerLimitStiffness=1e4  LowerLimitStiffnessUnits=N*m/deg  LowerLimitDamping=10  LowerLimitDampingUnits=N*m/(deg/s)  LowerLimitTransitionRegionWidth=0.1  LowerLimitTransitionRegionWidthUnits=deg  UpperLimitSpecify=on  UpperLimitBound=45  UpperLimitBoundUnits=deg  UpperLimitStiffness=1e4  UpperLimitStiffnessUnits=N*m/deg  UpperLimitDamping=10  UpperLimitDampingUnits=N*m/(deg/s)  UpperLimitTransitionRegionWidth=0.1  UpperLimitTransitionRegionWidthUnits=deg  PositionTargetSpecify=on  PositionTargetPriority=Low  PositionTargetValue=smiData.RevoluteJoint(6).Rz.Pos  PositionTargetValueUnits=deg  VelocityTargetSpecify=off  VelocityTargetPriority=High  VelocityTargetValue=0  VelocityTargetValueUnits=deg/s
  Mux1 : Mux  Inputs=7
  PS-Simulink Converter{1..7} (7 alike) : nesl_utility/PS-Simulink Converter  PhysicalDomain=network_engine_domain  SubClassName=ps_output  LeftPortType=input  RightPortType=output  PseudoPeriodic=off  Frequencies=[]  VectorFormat=1-D array  Unit=inherit  AffineConversion=off
  Revolute1 : sm_lib/Joints/Revolute Joint  JointMode=Normal  SenseConstraintForce=off  SenseConstraintForceX=off  SenseConstraintForceY=off  SenseConstraintForceZ=off  SenseConstraintTorque=off  SenseConstraintTorqueX=off  SenseConstraintTorqueY=off  SenseConstraintTorqueZ=off  SenseTotalForce=off  SenseTotalForceX=off  SenseTotalForceY=off  SenseTotalForceZ=off  SenseTotalTorque=off  SenseTotalTorqueX=off  SenseTotalTorqueY=off  SenseTotalTorqueZ=off  CompositeWrenchDir=FollowerOnBase  CompositeWrenchFrame=BaseFrame  EquilibriumPosition=0  EquilibriumPositionUnits=deg  SpringStiffness=0  SpringStiffnessUnits=N*m/deg  DampingCoefficient=0  DampingCoefficientUnits=N*m/(deg/s)  TorqueActuationMode=InputTorque  MotionActuationMode=ComputedMotion  SensePosition=on  SenseVelocity=off  SenseAcceleration=off  SenseTorqueForce=off  SenseLowerLimitTorqueForce=off  SenseUpperLimitTorqueForce=off  LowerLimitSpecify=on  LowerLimitBound=-25  LowerLimitBoundUnits=deg  LowerLimitStiffness=1e4  LowerLimitStiffnessUnits=N*m/deg  LowerLimitDamping=10  LowerLimitDampingUnits=N*m/(deg/s)  LowerLimitTransitionRegionWidth=0.1  LowerLimitTransitionRegionWidthUnits=deg  UpperLimitSpecify=on  UpperLimitBound=25  UpperLimitBoundUnits=deg  UpperLimitStiffness=1e4  UpperLimitStiffnessUnits=N*m/deg  UpperLimitDamping=10  UpperLimitDampingUnits=N*m/(deg/s)  UpperLimitTransitionRegionWidth=0.1  UpperLimitTransitionRegionWidthUnits=deg  PositionTargetSpecify=on  PositionTargetPriority=Low  PositionTargetValue=smiData.RevoluteJoint(4).Rz.Pos  PositionTargetValueUnits=deg  VelocityTargetSpecify=off  VelocityTargetPriority=High  VelocityTargetValue=0  VelocityTargetValueUnits=deg/s
  Revolute2 : sm_lib/Joints/Revolute Joint  JointMode=Normal  SenseConstraintForce=off  SenseConstraintForceX=off  SenseConstraintForceY=off  SenseConstraintForceZ=off  SenseConstraintTorque=off  SenseConstraintTorqueX=off  SenseConstraintTorqueY=off  SenseConstraintTorqueZ=off  SenseTotalForce=off  SenseTotalForceX=off  SenseTotalForceY=off  SenseTotalForceZ=off  SenseTotalTorque=off  SenseTotalTorqueX=off  SenseTotalTorqueY=off  SenseTotalTorqueZ=off  CompositeWrenchDir=FollowerOnBase  CompositeWrenchFrame=BaseFrame  EquilibriumPosition=0  EquilibriumPositionUnits=deg  SpringStiffness=0  SpringStiffnessUnits=N*m/deg  DampingCoefficient=0  DampingCoefficientUnits=N*m/(deg/s)  TorqueActuationMode=InputTorque  MotionActuationMode=ComputedMotion  SensePosition=on  SenseVelocity=off  SenseAcceleration=off  SenseTorqueForce=off  SenseLowerLimitTorqueForce=off  SenseUpperLimitTorqueForce=off  LowerLimitSpecify=on  LowerLimitBound=-25  LowerLimitBoundUnits=deg  LowerLimitStiffness=1e4  LowerLimitStiffnessUnits=N*m/deg  LowerLimitDamping=10  LowerLimitDampingUnits=N*m/(deg/s)  LowerLimitTransitionRegionWidth=0.1  LowerLimitTransitionRegionWidthUnits=deg  UpperLimitSpecify=on  UpperLimitBound=25  UpperLimitBoundUnits=deg  UpperLimitStiffness=1e4  UpperLimitStiffnessUnits=N*m/deg  UpperLimitDamping=10  UpperLimitDampingUnits=N*m/(deg/s)  UpperLimitTransitionRegionWidth=0.1  UpperLimitTransitionRegionWidthUnits=deg  PositionTargetSpecify=on  PositionTargetPriority=Low  PositionTargetValue=smiData.RevoluteJoint(4).Rz.Pos  PositionTargetValueUnits=deg  VelocityTargetSpecify=off  VelocityTargetPriority=High  VelocityTargetValue=0  VelocityTargetValueUnits=deg/s
  Simulink-PS Converter{1..7} (7 alike) : nesl_utility/Simulink-PS Converter  PhysicalDomain=network_engine_domain  SubClassName=ps_input  LeftPortType=input  RightPortType=output  PseudoPeriodic=off  Frequencies=[]  NoiseDistribution=none  NoiseParameters=[]  Unit=N*m  AffineConversion=off  FilteringAndDerivatives=provide  SimscapeFilterOrder=1  InputFilterTimeConstant=0.001  UdotUserProvided=0
  Yaw Guide to Hindfoot Base upper : sm_lib/Joints/Revolute Joint  JointMode=Normal  SenseConstraintForce=off  SenseConstraintForceX=off  SenseConstraintForceY=off  SenseConstraintForceZ=off  SenseConstraintTorque=off  SenseConstraintTorqueX=off  SenseConstraintTorqueY=off  SenseConstraintTorqueZ=off  SenseTotalForce=off  SenseTotalForceX=off  SenseTotalForceY=off  SenseTotalForceZ=off  SenseTotalTorque=off  SenseTotalTorqueX=off  SenseTotalTorqueY=off  SenseTotalTorqueZ=off  CompositeWrenchDir=FollowerOnBase  CompositeWrenchFrame=BaseFrame  EquilibriumPosition=0  EquilibriumPositionUnits=deg  SpringStiffness=0  SpringStiffnessUnits=N*m/deg  DampingCoefficient=0  DampingCoefficientUnits=N*m/(deg/s)  TorqueActuationMode=InputTorque  MotionActuationMode=ComputedMotion  SensePosition=on  SenseVelocity=off  SenseAcceleration=off  SenseTorqueForce=off  SenseLowerLimitTorqueForce=off  SenseUpperLimitTorqueForce=off  LowerLimitSpecify=on  LowerLimitBound=-40  LowerLimitBoundUnits=deg  LowerLimitStiffness=1e4  LowerLimitStiffnessUnits=N*m/deg  LowerLimitDamping=10  LowerLimitDampingUnits=N*m/(deg/s)  LowerLimitTransitionRegionWidth=0.1  LowerLimitTransitionRegionWidthUnits=deg  UpperLimitSpecify=on  UpperLimitBound=40  UpperLimitBoundUnits=deg  UpperLimitStiffness=1e4  UpperLimitStiffnessUnits=N*m/deg  UpperLimitDamping=10  UpperLimitDampingUnits=N*m/(deg/s)  UpperLimitTransitionRegionWidth=0.1  UpperLimitTransitionRegionWidthUnits=deg  PositionTargetSpecify=on  PositionTargetPriority=Low  PositionTargetValue=smiData.RevoluteJoint(3).Rz.Pos  PositionTargetValueUnits=deg  VelocityTargetSpecify=off  VelocityTargetPriority=High  VelocityTargetValue=0  VelocityTargetValueUnits=deg/s
  Yaw to Meta : sm_lib/Joints/Revolute Joint  JointMode=Normal  SenseConstraintForce=off  SenseConstraintForceX=off  SenseConstraintForceY=off  SenseConstraintForceZ=off  SenseConstraintTorque=off  SenseConstraintTorqueX=off  SenseConstraintTorqueY=off  SenseConstraintTorqueZ=off  SenseTotalForce=off  SenseTotalForceX=off  SenseTotalForceY=off  SenseTotalForceZ=off  SenseTotalTorque=off  SenseTotalTorqueX=off  SenseTotalTorqueY=off  SenseTotalTorqueZ=off  CompositeWrenchDir=FollowerOnBase  CompositeWrenchFrame=BaseFrame  EquilibriumPosition=0  EquilibriumPositionUnits=deg  SpringStiffness=0  SpringStiffnessUnits=N*m/deg  DampingCoefficient=0  DampingCoefficientUnits=N*m/(deg/s)  TorqueActuationMode=InputTorque  MotionActuationMode=ComputedMotion  SensePosition=on  SenseVelocity=off  SenseAcceleration=off  SenseTorqueForce=off  SenseLowerLimitTorqueForce=off  SenseUpperLimitTorqueForce=off  LowerLimitSpecify=on  LowerLimitBound=-25  LowerLimitBoundUnits=deg  LowerLimitStiffness=1e4  LowerLimitStiffnessUnits=N*m/deg  LowerLimitDamping=10  LowerLimitDampingUnits=N*m/(deg/s)  LowerLimitTransitionRegionWidth=0.1  LowerLimitTransitionRegionWidthUnits=deg  UpperLimitSpecify=on  UpperLimitBound=25  UpperLimitBoundUnits=deg  UpperLimitStiffness=1e4  UpperLimitStiffnessUnits=N*m/deg  UpperLimitDamping=10  UpperLimitDampingUnits=N*m/(deg/s)  UpperLimitTransitionRegionWidth=0.1  UpperLimitTransitionRegionWidthUnits=deg  PositionTargetSpecify=on  PositionTargetPriority=Low  PositionTargetValue=smiData.RevoluteJoint(5).Rz.Pos  PositionTargetValueUnits=deg  VelocityTargetSpecify=off  VelocityTargetPriority=High  VelocityTargetValue=0  VelocityTargetValueUnits=deg/s
  Conn1 : PMIOPort  Side=Left
  Conn2 : PMIOPort  Port=2  Side=Left
  Position : Outport
  wires:
  PS-Simulink Converter1/1 -> Mux1/3
  PS-Simulink Converter2/1 -> Mux1/2
  PS-Simulink Converter7/1 -> Mux1/1
  Demux/1 -> Simulink-PS Converter1/1
  PS-Simulink Converter6/1 -> Mux1/7
  PS-Simulink Converter5/1 -> Mux1/6
  PS-Simulink Converter4/1 -> Mux1/5
  PS-Simulink Converter3/1 -> Mux1/4
  Mux1/1 -> Position/1
  torque/1 -> Demux/1
  Demux/7 -> Simulink-PS Converter7/1
  Demux/6 -> Simulink-PS Converter6/1
  Demux/5 -> Simulink-PS Converter5/1
  Demux/4 -> Simulink-PS Converter4/1
  Demux/3 -> Simulink-PS Converter3/1
  Demux/2 -> Simulink-PS Converter2/1
  connections:
  HF Yaw Link to Yaw Guide/RConn2 -- PS-Simulink Converter1/LConn1
  Revolute1/RConn2 -- PS-Simulink Converter2/LConn1
  Revolute2/RConn2 -- PS-Simulink Converter7/LConn1
  Simulink-PS Converter3/RConn1 -- HF Yaw Link to Yaw Guide/LConn2
  Simulink-PS Converter2/RConn1 -- Revolute1/LConn2
  Revolute2/LConn2 -- Simulink-PS Converter1/RConn1
  Hindfoot Yaw Subsystem/LConn1 -- Revolute2/RConn1
  Simulink-PS Converter4/RConn1 -- Yaw Guide to Hindfoot Base upper/LConn2
  Yaw Guide to Hindfoot Base upper/RConn2 -- PS-Simulink Converter3/LConn1
  Forefoot Subsystem/LConn3 -- Yaw to Meta/LConn1
  Forefoot Subsystem/RConn1 -- Coupling to Yaw Link/RConn1
  Simulink-PS Converter5/RConn1 -- Hindfoot to Roll Link/LConn2
  Yaw to Meta/RConn2 -- PS-Simulink Converter5/LConn1
  Coupling to Yaw Link/RConn2 -- PS-Simulink Converter6/LConn1
  Simulink-PS Converter7/RConn1 -- Coupling to Yaw Link/LConn2
  Revolute1/LConn1 -- Conn2/RConn1
  Forefoot Subsystem/LConn2 -- Coupling to Yaw Link/LConn1
  Simulink-PS Converter6/RConn1 -- Yaw to Meta/LConn2
  Forefoot Subsystem/RConn2 -- Yaw to Meta/RConn1
  Hindfoot Yaw Subsystem/LConn2 -- HF Yaw Link to Yaw Guide/LConn1
  Hindfoot Yaw Subsystem/RConn2 -- HF Yaw Link to Yaw Guide/RConn1
  Conn1/RConn1 -- Revolute2/LConn1
  Revolute1/RConn1 -- Hindfoot Pitch Subsystem/LConn1
  Hindfoot to Roll Link/RConn1 -- Forefoot Subsystem/LConn1
  Hindfoot to Roll Link/LConn1 -- Hindfoot Base Subsystem/RConn1
  Hindfoot to Roll Link/RConn2 -- PS-Simulink Converter4/LConn1
  Yaw Guide to Hindfoot Base upper/RConn1 -- Hindfoot Base Subsystem/LConn1
  Yaw Guide to Hindfoot Base upper/LConn1 -- Hindfoot Yaw Subsystem/RConn1

== system IK_Six_DOF_assembly2/Robot1/Thigh//Slider Subsystem1 ==
  x4_1_Slider_Link_1_RIGID : Subsystem
  x4_3_Thigh_Link_1_RIGID : Subsystem
  F1 : PMIOPort  Side=Left
  F2 : PMIOPort  Port=2  Side=Right
  connections:
  F2/RConn1 -- x4_1_Slider_Link_1_RIGID/LConn2
  F1/RConn1 -- x4_1_Slider_Link_1_RIGID/LConn1
  x4_1_Slider_Link_1_RIGID/LConn3 -- x4_3_Thigh_Link_1_RIGID/LConn1

== system IK_Six_DOF_assembly2/Robot1/Thigh//Slider Subsystem2 ==
  x4_1_Slider_Link_2_RIGID : Subsystem
  x4_3_Thigh_Link_2_RIGID : Subsystem
  F : PMIOPort  Side=Left
  connections:
  F/RConn1 -- x4_1_Slider_Link_2_RIGID/LConn2
  x4_1_Slider_Link_2_RIGID/LConn1 -- x4_3_Thigh_Link_2_RIGID/LConn1

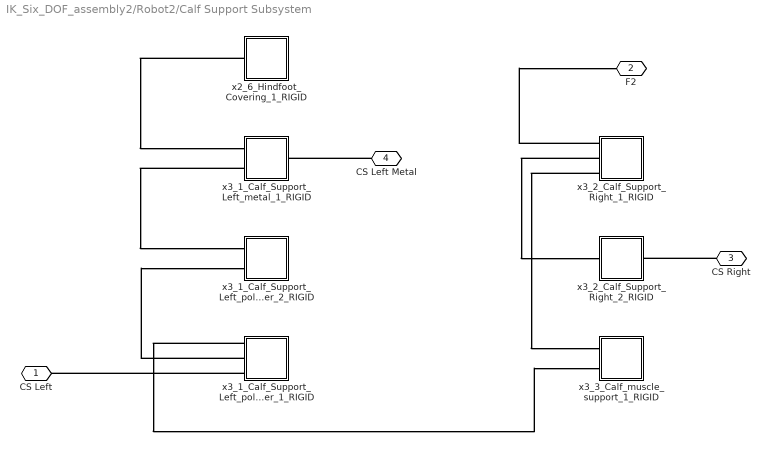
== system IK_Six_DOF_assembly2/Robot2/Calf Support Subsystem ==
  x2_6_Hindfoot_Covering_1_RIGID : Subsystem
  x3_1_Calf_Support_Left_metal_1_RIGID : Subsystem
  x3_1_Calf_Support_Left_poly_upper_1_RIGID : Subsystem
  x3_1_Calf_Support_Left_poly_upper_2_RIGID : Subsystem
  x3_2_Calf_Support_Right_1_RIGID : Subsystem
  x3_2_Calf_Support_Right_2_RIGID : Subsystem
  x3_3_Calf_muscle_support_1_RIGID : Subsystem
  "CS Left " : PMIOPort  Side=Left
  F2 : PMIOPort  Port=2  Side=Left
  CS Right : PMIOPort  Port=3  Side=Right
  CS Left Metal : PMIOPort  Port=4  Side=Right
  connections:
  x2_6_Hindfoot_Covering_1_RIGID/LConn1 -- x3_1_Calf_Support_Left_metal_1_RIGID/LConn1
  x3_2_Calf_Support_Right_1_RIGID/LConn1 -- F2/RConn1
  x3_1_Calf_Support_Left_poly_upper_1_RIGID/LConn1 -- x3_3_Calf_muscle_support_1_RIGID/LConn2
  x3_2_Calf_Support_Right_1_RIGID/LConn2 -- x3_2_Calf_Support_Right_2_RIGID/LConn1
  CS Left Metal/RConn1 -- x3_1_Calf_Support_Left_metal_1_RIGID/RConn1
  x3_1_Calf_Support_Left_metal_1_RIGID/LConn2 -- x3_1_Calf_Support_Left_poly_upper_2_RIGID/LConn1
  x3_2_Calf_Support_Right_1_RIGID/LConn3 -- x3_3_Calf_muscle_support_1_RIGID/LConn1
  x3_1_Calf_Support_Left_poly_upper_1_RIGID/LConn2 -- x3_1_Calf_Support_Left_poly_upper_2_RIGID/LConn2
  CS Right/RConn1 -- x3_2_Calf_Support_Right_2_RIGID/RConn1
  x3_1_Calf_Support_Left_poly_upper_1_RIGID/LConn3 -- "CS Left "/RConn1

== system IK_Six_DOF_assembly2/Robot2/Initializer ==
  MechanismConfiguration : sm_lib/Utilities/Mechanism Configuration  UniformGravity=Constant  GravityVector=[0 0 -9.80665]  GravityUnits=m/s^2  LinearizationDelta=0.001  JointModeTransitionNonlinearIterations=2
  Solver Configuration : nesl_utility/Solver Configuration  PhysicalDomain=network_engine_domain  SubClassName=solver  LeftPortType=input  RightPortType=generic  Tones=[]  Harmonics=[]  SimulateNoise=off  Profile=off  UseLocalSampling=off  EnableSwitchedLinearOptims=on  FrequencyDomain=off  UseCCode=off  RelTol=0.001  AbsTol=1e-06  MinStep=1e-09  ToWorkspace=off  RevertToSquareIcSolve=off  NumHomotopyIterations=100  PhasorMode=off  PhasorModeNumHarmonics=1  ConsistencySolver=NEWTON_FTOL  IndexReductionMethod=DerivativeReplacement  DoDC=off  ResidualTolerance=1e-09  ConsistencyTolSource=GLOBAL  ConsistencyAbsTol=0.001  ConsistencyRelTol=0.001  ConsistencyTolFactor=0.001  UseLocalSolver=off  LocalSolverChoice=NE_BACKWARD_EULER_ADVANCER  ResolveIndetEquations=on  FunctionEvalNumThread=1  LocalSolverSampleTime=0.001  DoFixedCost=off  MaxNonlinIter=3  MaxModeIter=2  ComputeImpulses=off  ImpulseIterations=2  LinearAlgebra=auto  LinearAlgebraNumThread=0  EquationFormulation=NE_TIME_EF  DelaysMemoryBudget=1024  AutomaticFiltering=on  FilteringTimeConstant=0.001  PartitionStorageMethod=AS_NEEDED  PartitionMemoryBudget=1024  PartitionMethod=ROBUST
  Transform : sm_lib/Frames and Transforms/Rigid Transform  TranslationMethod=Cartesian  TranslationStandardOffset=0  TranslationLengthUnit=in  TranslationStandardAxis=+Z  TranslationCartesianOffset=smiData.RigidTransform(63).translation  TranslationROffset=0  TranslationROffsetUnits=m  TranslationZOffset=0  TranslationZOffsetUnits=m  TranslationThetaOffset=0  TranslationThetaOffsetUnits=deg  RotationMethod=ArbitraryAxis  RotationAngleUnits=rad  RotationStandardAxis=+Z  RotationAngle=smiData.RigidTransform(63).angle  RotationArbitraryAxis=smiData.RigidTransform(63).axis  FollAlignAxisA=+X  BaseAlignAxisA=+Y  FollAlignAxisB=+Y  BaseAlignAxisB=+Z  RotationSequenceAxes=FollowerAxes  RotationSequence=XYX  RotationSequenceAngles=[0 0 0]  RotationSequenceAnglesUnits=deg  RotationMatrix=[1 0 0; 0 1 0; 0 0 1]  Quaternion=[1 0 0 0]
  World : sm_lib/Frames and Transforms/World Frame
  F2 : PMIOPort  Side=Right
  connections:
  Transform/LConn1 -- Solver Configuration/RConn1 -- MechanismConfiguration/RConn1 -- World/RConn1
  Transform/RConn1 -- F2/RConn1
